simulink model "system"  (R2020a)
settings: Solver=VariableStepAuto  StartTime=0.0  StopTime=360  RelTol=1e-3
libraries: simulink x1, simulink_extras x1
settings Model: Creator=chooxuanwing  LastModifiedBy=chooxuanwing

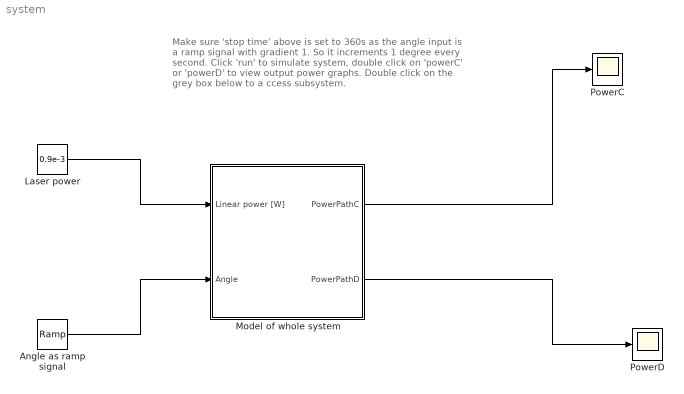
== system system ==
  note: Make sure 'stop time' above is set to 360s as the angle input is a ramp signal with gradient 1.
      | So it increments 1 degree every second.
      |
      | Click 'run' to simulate system, double click on 'powerC' or 'powerD' to view output power graphs.
      |
      | Double click on the grey box below to a
      | ccess subsystem.
  Angle as ramp signal : simulink/Sources/Ramp  slope=1  start=0  InitialOutput=0
  Laser power : Constant  Value=0.9e-3
  Model of whole system : Subsystem
  PowerC : Scope
  PowerD : Scope
  wires:
  Laser power/1 -> Model of whole system/1(Linear power [W])
  Angle as ramp signal/1 -> Model of whole system/2(Angle)
  Model of whole system/1(PowerPathC) -> PowerC/1
  Model of whole system/2(PowerPathD) -> PowerD/1

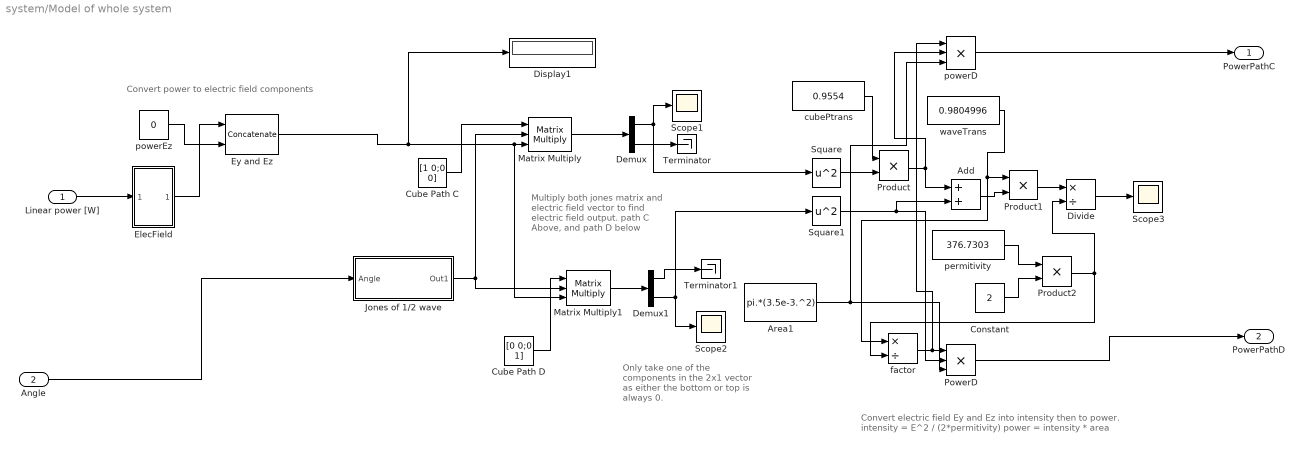
== system system/Model of whole system ==
  note: Only take one of the components in the 2x1 vector as either the bottom or top is always 0.
  note: Convert electric field Ey and Ez into intensity then to power.
      | intensity = E^2 / (2*permitivity)
      | power = intensity * area
  note: Multiply both jones matrix and electric field vector to find electric field output.
      |
      | path C Above, and path D below
  note: Convert power to electric field components
  Linear power [W] : Inport
  Angle : Inport  Port=2
  Add : Sum
  Area1 : Constant  Value=pi.*(3.5e-3.^2)
  Constant : Constant  Value=2
  Cube Path C : Constant  Value=[1 0;0 0]
  Cube Path D : Constant  Value=[0 0;0 1]
  Demux : Demux  Outputs=2
  Demux1 : Demux  Outputs=2
  Display1 : Display
  Divide : Product  Inputs=*/
  ElecField : Subsystem
  Ey and Ez : Concatenate  Mode=Multidimensional array
  Jones of 1/2 wave : Subsystem
  Matrix Multiply : Product  Inputs=3  Multiplication=Matrix(*)
  Matrix Multiply1 : Product  Inputs=3  Multiplication=Matrix(*)
  PowerD : Product  Inputs=3
  Product : Product
  Product1 : Product
  Product2 : Product
  Scope1 : Scope
  Scope2 : Scope
  Scope3 : Scope
  Square : Math  Operator=square  SaturateOnIntegerOverflow=on
  Square1 : Math  Operator=square  SaturateOnIntegerOverflow=on
  Terminator : Terminator
  Terminator1 : Terminator
  cubePtrans : Constant  Value=0.9554
  factor : Product  Inputs=*/
  permitivity : Constant  Value=376.7303
  powerD : Product  Inputs=3
  powerEz : Constant  Value=0
  waveTrans : Constant  Value=0.9804996
  PowerPathC : Outport
  PowerPathD : Outport  Port=2
  wires:
  factor/1 -> powerD/1, PowerD/1
  Angle/1 -> Jones of 1/2 wave/1(Angle)
  cubePtrans/1 -> Product/1
  Add/1 -> Product1/2
  Divide/1 -> Scope3/1
  waveTrans/1 -> factor/1, Product1/1
  Product2/1 -> factor/2, Divide/2
  Square1/1 -> PowerD/2, Add/2
  Area1/1 -> powerD/3, PowerD/3
  powerEz/1 -> Ey and Ez/2
  Product1/1 -> Divide/1
  ElecField/1(Out1) -> Ey and Ez/1
  Constant/1 -> Product2/2
  Linear power [W]/1 -> ElecField/1(In1)
  Square/1 -> Product/2
  PowerD/1 -> PowerPathD/1
  Jones of 1/2 wave/1(Out1) -> Matrix Multiply1/2, Matrix Multiply/2
  Demux/2 -> Terminator/1
  Product/1 -> powerD/2, Add/1
  Cube Path C/1 -> Matrix Multiply/1
  Demux/1 -> Square/1, Scope1/1
  Cube Path D/1 -> Matrix Multiply1/1
  Demux1/2 -> Square1/1, Scope2/1
  powerD/1 -> PowerPathC/1
  Demux1/1 -> Terminator1/1
  Matrix Multiply1/1 -> Demux1/1
  Ey and Ez/1 -> Display1/1, Matrix Multiply1/3, Matrix Multiply/3
  permitivity/1 -> Product2/1
  Matrix Multiply/1 -> Demux/1

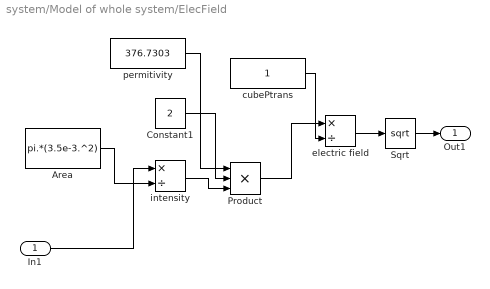
== system system/Model of whole system/ElecField ==
  In1 : Inport
  Area : Constant  Value=pi.*(3.5e-3.^2)
  Constant1 : Constant  Value=2
  Product : Product  Inputs=3
  Sqrt : Sqrt  SaturateOnIntegerOverflow=on
  cubePtrans : Constant
  electric field : Product  Inputs=*/
  intensity : Product  Inputs=*/
  permitivity : Constant  Value=376.7303
  Out1 : Outport
  wires:
  In1/1 -> intensity/1
  Constant1/1 -> Product/2
  permitivity/1 -> Product/1
  intensity/1 -> Product/3
  Product/1 -> electric field/1
  electric field/1 -> Sqrt/1
  cubePtrans/1 -> electric field/2
  Area/1 -> intensity/2
  Sqrt/1 -> Out1/1

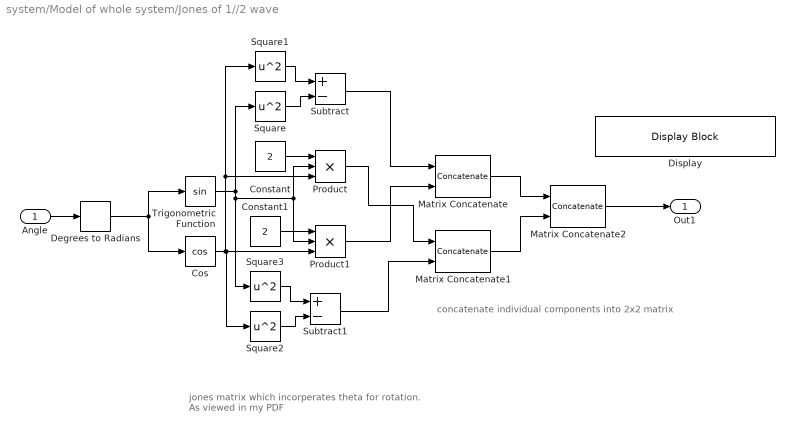
== system system/Model of whole system/Jones of 1//2 wave ==
  note: concatenate individual components into 2x2 matrix
  note: jones matrix which incorperates theta for rotation.
      | As viewed in my PDF
  Angle : Inport
  Constant : Constant  Value=2
  Constant1 : Constant  Value=2
  Cos : Trigonometry  Operator=cos
  Degrees to Radians : simulink_extras/Transformations/Degrees to Radians
  Display : DisplayBlock  LabelPosition=Hide  Format=short  Transparency=1
  Matrix Concatenate : Concatenate  Mode=Multidimensional array  ConcatenateDimension=2
  Matrix Concatenate1 : Concatenate  Mode=Multidimensional array  ConcatenateDimension=2
  Matrix Concatenate2 : Concatenate  Mode=Multidimensional array
  Product : Product  Inputs=3
  Product1 : Product  Inputs=3
  Square{,1..3} (4 alike) : Math  Operator=square  SaturateOnIntegerOverflow=on
  Subtract : Sum  Inputs=+-
  Subtract1 : Sum  Inputs=+-
  Trigonometric Function : Trigonometry
  Out1 : Outport
  wires:
  Angle/1 -> Degrees to Radians/1
  Degrees to Radians/1 -> Cos/1, Trigonometric Function/1
  Trigonometric Function/1 -> Square/1, Square3/1, Product1/2, Product/2
  Square1/1 -> Subtract/1
  Square/1 -> Subtract/2
  Constant/1 -> Product/1
  Constant1/1 -> Product1/1
  Square2/1 -> Subtract1/2
  Square3/1 -> Subtract1/1
  Cos/1 -> Square2/1, Product1/3, Product/3, Square1/1
  Subtract/1 -> Matrix Concatenate/1
  Product1/1 -> Matrix Concatenate/2
  Product/1 -> Matrix Concatenate1/1
  Subtract1/1 -> Matrix Concatenate1/2
  Matrix Concatenate/1 -> Matrix Concatenate2/1
  Matrix Concatenate1/1 -> Matrix Concatenate2/2
  Matrix Concatenate2/1 -> Out1/1
